simulink model "chapter4_jd"  (R2016b)
settings: Solver=VariableStepAuto  StartTime=0.0  StopTime=10.0  RelTol=1e-3
PreLoadFcn:
  | load throttle_input;
  | etc_plant_data;
  | % etc_plant_data_limit;
undefined symbols (not defined in the file): Cs, J, Kd, Ks, theta_eq
settings Model: Creator=training-ah  LastModifiedBy=training-ah
settings DataIOCC: ExternalInput=[t, duty, direction]  LoadExternalInput=on  SaveFormat=Array

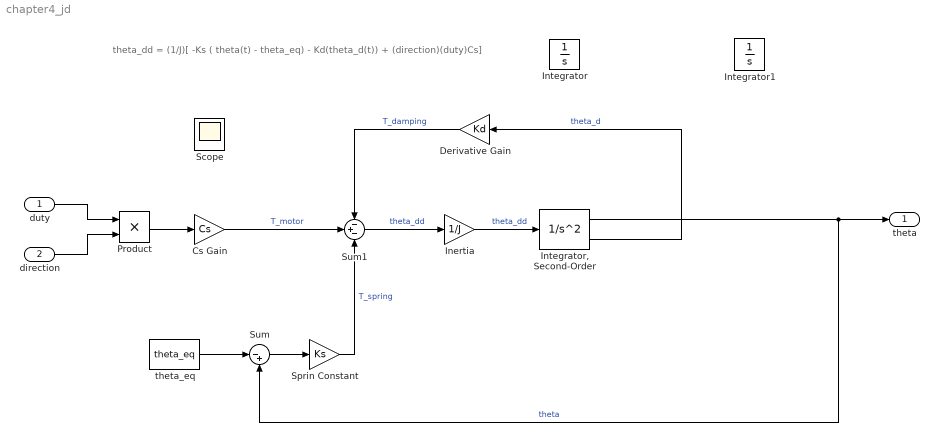
== system chapter4_jd ==
  note: theta_dd = (1/J)[ -Ks ( theta(t) - theta_eq) - Kd(theta_d(t)) + (direction)(duty)Cs]
  duty : Inport
  direction : Inport  Port=2
  Cs Gain : Gain  Gain=Cs
  Derivative Gain : Gain  Gain=Kd
  "Inertia " : Gain  Gain=1/J
  Integrator : Integrator
  "Integrator, Second-Order" : SecondOrderIntegrator  ICX=pi/6  LimitX=on  UpperLimitX=pi/2  LowerLimitX=0  ReinitDXDTwhenXreachesSaturation=on
  Integrator1 : Integrator  InitialCondition=pi/6  LimitOutput=on  UpperSaturationLimit=pi/2  LowerSaturationLimit=0
  Product : Product
  Sprin Constant : Gain  Gain=Ks
  Sum : Sum  Inputs=|-+
  Sum1 : Sum  Inputs=-+-
  "theta_eq " : Constant  Value=theta_eq
  theta : Outport
  Scope : Scope
  wires:
  "Inertia "/1 -> "Integrator, Second-Order"/1  "theta_dd"
  "Integrator, Second-Order"/1 -> Sum/2, theta/1  "theta"
  Derivative Gain/1 -> Sum1/1  "T_damping"
  duty/1 -> Product/1
  direction/1 -> Product/2
  Product/1 -> Cs Gain/1
  Cs Gain/1 -> Sum1/2  "T_motor"
  "theta_eq "/1 -> Sum/1
  Sum/1 -> Sprin Constant/1
  Sprin Constant/1 -> Sum1/3  "T_spring"
  Sum1/1 -> "Inertia "/1  "theta_dd"
  "Integrator, Second-Order"/2 -> Derivative Gain/1  "theta_d"
